simulink model "ControlledUnicycleAndDifferentialDrive"  (R2024b)
settings: Solver=VariableStepAuto  StartTime=0.0  StopTime=10.0  RelTol=1e-3
values from neighbouring files (symbols this model uses):
  A = [ k1*v*cos(theta) 0 -v*sin(theta) ... (first row only)    [SimRun.m]
  B = [  0    0 ... (first row only)    [SimRun.m]
  C = [1 0 0 ... (first row only)    [SimRun.m]
  D = [0 0 ... (first row only)    [SimRun.m]
  IC = [-1 1 pi/4]    [SimRun.m]
  L = 0.5    [SimRun.m]
  R = 0.1    [SimRun.m]
settings Model: Creator=elija  LastModifiedBy=elija

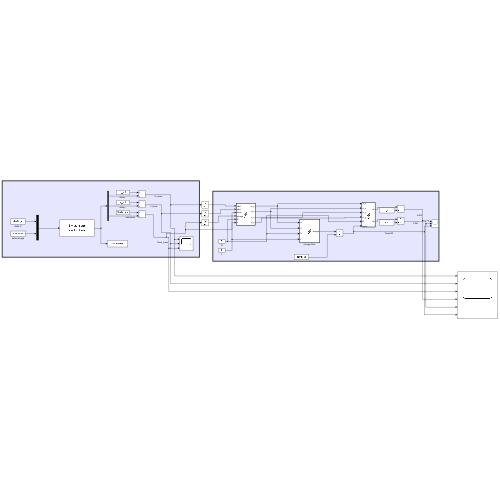
[thumbnail: Simulink's stored preview of the top-level diagram]
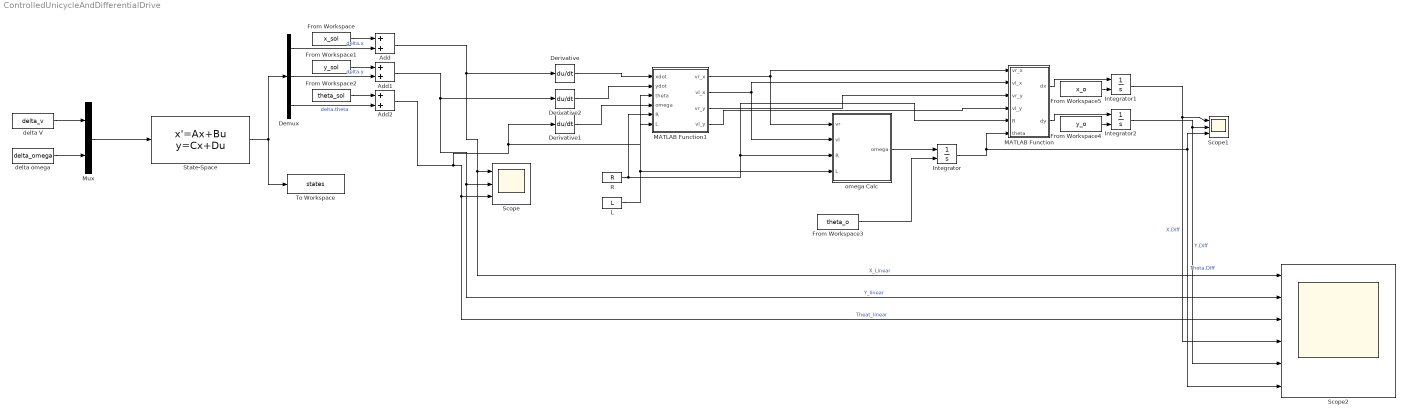
== system ControlledUnicycleAndDifferentialDrive ==
  Add : Sum
  Add1 : Sum
  Add2 : Sum
  Demux : Demux  Outputs=3
  Derivative : Derivative
  Derivative1 : Derivative
  Derivative2 : Derivative
  From Workspace : FromWorkspace  VariableName=x_sol
  From Workspace1 : FromWorkspace  VariableName=y_sol
  From Workspace2 : FromWorkspace  VariableName=theta_sol
  From Workspace3 : FromWorkspace  VariableName=theta_o
  From Workspace4 : FromWorkspace  VariableName=y_o
  From Workspace5 : FromWorkspace  VariableName=x_o
  Integrator : Integrator  InitialConditionSource=external
  Integrator1 : Integrator  InitialConditionSource=external
  Integrator2 : Integrator  InitialConditionSource=external
  L : Constant  Value=L
  MATLAB Function : MATLAB Function  TreatAsAtomicUnit=on
  MATLAB Function1 : MATLAB Function  TreatAsAtomicUnit=on
  Mux : Mux  Inputs=2
  R : Constant  Value=R
  Scope : Scope  NumInputPorts=3
  Scope1 : Scope  NumInputPorts=3
  Scope2 : Scope  NumInputPorts=6
  State-Space : StateSpace  A=A  B=B  C=C  D=D  InitialCondition=IC
  To Workspace : ToWorkspace  VariableName=states  SaveFormat=Timeseries  SampleTime=-1
  delta V : FromWorkspace  VariableName=delta_v
  delta omega : FromWorkspace  VariableName=delta_omega
  omega Calc : MATLAB Function  TreatAsAtomicUnit=on
  wires:
  From Workspace2/1 -> Add2/1
  Demux/3 -> Add2/2  "delta.theta"
  Integrator2/1 -> Scope2/5, Scope1/2  "Y.Diff"
  Integrator1/1 -> Scope2/4, Scope1/1  "X.Diff"
  From Workspace/1 -> Add/1
  MATLAB Function1/1(vr_x) -> omega Calc/1(vr), MATLAB Function/1(vr_x)
  MATLAB Function1/2(vl_x) -> omega Calc/2(vl), MATLAB Function/2(vl_x)
  R/1 -> MATLAB Function1/5(R), MATLAB Function/5(R), omega Calc/3(R)
  MATLAB Function/1(dx) -> Integrator1/1
  L/1 -> MATLAB Function1/6(L), omega Calc/4(L)
  MATLAB Function/2(dy) -> Integrator2/1
  From Workspace3/1 -> Integrator/2
  Integrator/1 -> Scope1/3, Scope2/6, MATLAB Function/6(theta)  "Theta.Diff"
  Add/1 -> Scope2/1, Scope/1, Derivative/1  "X_Linear"
  From Workspace1/1 -> Add1/1
  Demux/2 -> Add1/2  "delta.y"
  From Workspace5/1 -> Integrator1/2
  Add1/1 -> Scope2/2, Scope/2, Derivative2/1  "Y_linear"
  Derivative/1 -> MATLAB Function1/1(xdot)
  Add2/1 -> Derivative1/1, MATLAB Function1/3(theta), Scope2/3, Scope/3  "Theat_linear"
  delta V/1 -> Mux/1
  Demux/1 -> Add/2  "delta.x"
  delta omega/1 -> Mux/2
  omega Calc/1(omega) -> Integrator/1
  From Workspace4/1 -> Integrator2/2
  Mux/1 -> State-Space/1
  State-Space/1 -> To Workspace/1, Demux/1
  Derivative1/1 -> MATLAB Function1/4(omega)
  Derivative2/1 -> MATLAB Function1/2(ydot)
  MATLAB Function1/3(vr_y) -> MATLAB Function/3(vr_y)
  MATLAB Function1/4(vl_y) -> MATLAB Function/4(vl_y)

== matlab function ControlledUnicycleAndDifferentialDrive/omega Calc ==
  data: vr input; omega output; vl input; R input; L input
function omega = fcn(vr,vl,R,L)
omega = (R./L).*(vr-vl);
end

== matlab function ControlledUnicycleAndDifferentialDrive/MATLAB Function ==
  data: dx output; dy output; vr_x input; vl_x input; vr_y input; vl_y input; R input; theta input
function [dx,dy] = fcn(vr_x,vl_x,vr_y,vl_y,R,theta)

dy = (R./2).*(vr_y-vl_y).*sin(theta);
dx = (R./2).*(vr_x+-vl_x).*cos(theta);

end

== matlab function ControlledUnicycleAndDifferentialDrive/MATLAB Function1 ==
  data: xdot input; ydot input; vr_x output; theta input; omega input; R input; vl_x output; L input; vr_y output; vl_y output
function [vr_x,vl_x,vr_y,vl_y] = fcn(xdot,ydot,theta,omega,R,L)

vx = xdot./cos(theta);
vr_x = (2.*vx+omega*L)/(2*R);
vl_x = (2.*vx-omega*L)/(2*R);

vy = ydot./cos(theta);
vr_y = (2.*vy+omega*L)/(2*R);
vl_y = (2.*vy-omega*L)/(2*R);
end
